simulink model "ekf_soc_estimator"  (R2023b)
settings: Solver=FixedStepDiscrete  StartTime=0.0  StopTime=10.0  RelTol=1e-3  EnableMultiTasking=on
InitFcn:
  | startup_soc_simulink_model;
values from neighbouring files (symbols this model uses):
  params_struct = rmfield(params_struct, {'ocv_fun', 'ocv_grad'})    [startup_soc_simulink_model.m]
settings Model: Creator=aryan  LastModifiedBy=aryan
settings SolverCC: PositivePriorityOrder=on  AutoInsertRateTranBlk=on
settings DataIOCC: SaveOutput=off  SaveTime=off
settings OptimizationCC: DefaultParameterBehavior=Inlined  UseDivisionForNetSlopeComputation=on  GainParamInheritBuiltInType=on  UseFloatMulNetSlope=on  InlineInvariantSignals=on  PassReuseOutputArgsAs=Individual arguments  ZeroExternalMemoryAtStartup=off  ZeroInternalMemoryAtStartup=off  NoFixptDivByZeroProtection=on  EfficientFloat2IntCast=on  LifeSpan=1  MaxStackSize=64  OptimizeBlockOrder=speed  DifferentSizesBufferReuse=on  EfficientTunableParamExpr=on
settings DebuggingCC: ParameterTunabilityLossMsg=error  BusObjectLabelMismatch=error
settings HardwareCC: ProdBitPerPointer=32  ProdBitPerSizeT=32  ProdBitPerPtrDiffT=32  ProdLargestAtomicInteger=Long  ProdLargestAtomicFloat=Double  ProdWordSize=32  ProdLongLongMode=on  ProdHWDeviceType=ARM Compatible->ARM Cortex-M
settings SFSimCC: MATLABDynamicMemAlloc=off
settings RTWCC: Description=Embedded Coder  SystemTargetFile=ert.tlc  TLCOptions=-p0  GenCodeOnly=on  TemplateMakefile=ert_default_tmf  GenerateReport=on  RTWVerbose=off  Toolchain=GNU Tools for ARM Embedded Processors  IncludeHyperlinkInReport=on  LaunchReport=on
settings CodeAppCC: ForceParamTrailComments=on  IgnoreCustomStorageClasses=off  OperatorAnnotations=on  SimulinkDataObjDesc=on  SFDataObjDesc=on  CustomSymbolStrGlobalVar=rt$N$M  CustomSymbolStrType=$N$M  CustomSymbolStrFcn=$N$M$F  CustomSymbolStrMacro=$N$M  InsertBlockDesc=on
settings ERTTargetCC: TargetLangStandard=C99 (ISO)  CodeReplacementLibrary=ARM Cortex-M  IncludeMdlTerminateFcn=off  CombineSignalStateStructs=on  SupportAbsoluteTime=off  SupportComplex=off  SupportNonInlinedSFcns=on  ExtModeTransport=3  ExtModeStaticAlloc=on  ExtModeStaticAllocSize=2048  ExtModeMexFile=ext_xcp  ExtModeIntrfLevel=Level2 - Open  InlinedParameterPlacement=NonHierarchical  RootIOFormat=Structure reference  ERTCustomFileTemplate=example_file_process.tlc  ERTFilePackagingFormat=CompactWithDataFile

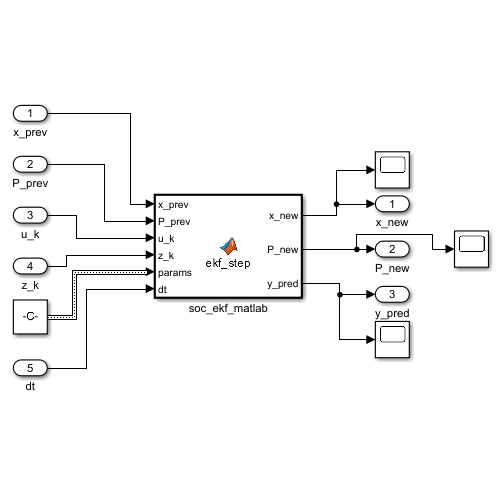
[thumbnail: Simulink's stored preview of the top-level diagram]
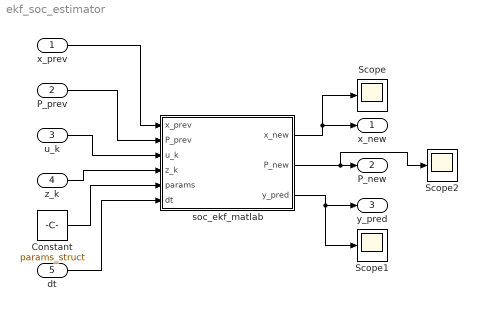
== system ekf_soc_estimator ==
  x_prev : Inport
  P_prev : Inport  Port=2
  u_k : Inport  Port=3
  z_k : Inport  Port=4
  dt : Inport  Port=5
  Constant : Constant  Value=params_struct  OutDataTypeStr=Bus: battery_bus
  Scope : Scope
  Scope1 : Scope
  Scope2 : Scope
  soc_ekf_matlab : MATLAB Function  TreatAsAtomicUnit=on
  x_new : Outport
  P_new : Outport  Port=2
  y_pred : Outport  Port=3
  wires:
  x_prev/1 -> soc_ekf_matlab/1(x_prev)
  P_prev/1 -> soc_ekf_matlab/2(P_prev)
  u_k/1 -> soc_ekf_matlab/3(u_k)
  z_k/1 -> soc_ekf_matlab/4(z_k)
  Constant/1 -> soc_ekf_matlab/5(params)
  dt/1 -> soc_ekf_matlab/6(dt)
  soc_ekf_matlab/1(x_new) -> Scope/1, x_new/1
  soc_ekf_matlab/2(P_new) -> Scope2/1, P_new/1
  soc_ekf_matlab/3(y_pred) -> Scope1/1, y_pred/1

== matlab function ekf_soc_estimator/soc_ekf_matlab ==
  data: x_prev input double size=[2 1]; x_new output double size=[2 1]; P_prev input double size=[2 2]; u_k input double size=1; z_k input double size=1; params input Bus: battery_bus; dt input double size=1; P_new output double size=[2 2]; y_pred output double size=1
% =========================================================================
% @file    ekf_step.m
% @brief   One Extended Kalman Filter iteration for battery SOC estimation
% @date    2025-09-07
% @author  Midnight Sun Team #24 - MSXVI
%
% =========================================================================
% FUNCTION DESCRIPTION
% =========================================================================
% Performs a single EKF cycle (predict + update) for a 2-state battery model
%
% -------------------------------------------------------------------------
% INPUTS:
%   x_prev  : double [2x1]
%       Previous state estimate [SOC; Vrc]
%   P_prev  : double [2x2]
%       Previous error covariance matrix
%   u_k     : double [scalar]
%       Current input (battery current, Amperes)
%   z_k     : double [scalar]
%       Current measurement (terminal voltage, Volts)
%   params  : struct
%       Battery model parameters
%   dt      : double [scalar]
%       Sampling time step (seconds)
%
% OUTPUTS:
%   x_new   : double [2x1]
%       Updated state estimate [SOC; Vrc]
%   P_new   : double [2x2]
%       Updated error covariance matrix
%   y_pred  : double [scalar]
%       Predicted measurement (terminal voltage, Volts)
%
% =========================================================================

function [x_new, P_new, y_pred] = ekf_step(x_prev, P_prev, u_k, z_k, params, dt) %#codegen
    % =========================================================================
    % NOISE COVARIANCE SETUP
    %
    % Process noise Q: How much we trust our battery model
    % Measurement noise R: How much we trust our voltage sensor
    % =========================================================================
    if isfield(params,'Q_proc')
        Q = params.Q_proc;                         % Use provided process noise
    else
        Q = single([1e-6, 0; 0, 1e-5]);            % Default: SOC very certain, Vrc less certain
    end
    
    if isfield(params,'R_meas')
        R = params.R_meas;                         % Use provided measurement noise
    else
        R = single(1e-3);
    end

    x_new = zeros(2,1);
    P_new = zeros(2,2);
    y_pred = 0;

    % =========================================================================
    % PREDICT STEP
    %
    % Use the battery state space model to predict where we'll be next
    % =========================================================================
    
    % Predict the next state using our battery model
    x_pred = ssm_state_update(x_prev, u_k, params, dt);
    x_pred(1) = clamp01(x_pred(1));

    % Get the linearized state transition matrix (Jacobian)
    Fd = ssm_state_jacobian(x_prev, u_k, params, dt);
    
    % Predict how uncertain we are about our prediction
    P_pred = Fd * P_prev * Fd' + Q;

    % =========================================================================
    % UPDATE STEP  
    %
    % Use the voltage measurement to correct our prediction
    % =========================================================================
    
    % Get the measurement sensitivity matrix (how voltage depends on states)
    H = ssm_output_jacobian(x_pred, u_k, params); % [dV/dSOC, dV/dVrc] = [OCV_slope, -1]

    % Predict what voltage we should see given our state prediction
    y_pred = ssm_output_fn(x_pred, u_k, params);  % V_terminal = OCV(SOC) - R0*I - Vrc

    % Calculate the innovation (how wrong our prediction was)
    voltage_error = z_k - y_pred;                 % Actual voltage - predicted voltage
    
    % Calculate innovation covariance (total uncertainty in the measurement space)
    measurement_uncertainty  = H * P_pred * H' + R;
    
    % Calculate Kalman gain (how much to trust the measurement vs prediction)
    kalman_gain = (P_pred * H') / measurement_uncertainty;  % Higher gain = trust measurement more
    
    % Update state estimate using the measurement
    x_new = x_pred + kalman_gain * voltage_error; % Blend prediction with measurement
    x_new(1) = clamp01(x_new(1));                 % Keep SOC physically reasonable
    
    % Update uncertainty using Joseph form (numerically stable)
    I2 = eye(2,'like',P_pred);                    % 2x2 identity matrix
    P_new = (I2 - kalman_gain * H) * P_pred * (I2 - kalman_gain * H)' + kalman_gain * R * kalman_gain';
end
